simulink model "Analisis_dos_tanques"  (R2019a)
settings: Solver=VariableStepAuto  StartTime=0.0  StopTime=8000  RelTol=1e-3
values from neighbouring files (symbols this model uses):
  A1 = 95.5200    (= 95.52)    [Cluster_Discrimin.m]
  A2 = 64    [Cluster_Discrimin.m]
  k1 = 0.95800    (= 0.958)    [Cluster_Discrimin.m]
  k2 = 1.363500    (= 1.3635)    [Cluster_Discrimin.m]
undefined symbols (not defined in the file or in its folder): errortub, perturbacion, perturbacion2
settings Model: Creator=jalil  LastModifiedBy=david
settings DebuggingCC: ArithmeticOperatorsInVariantConditions=warning

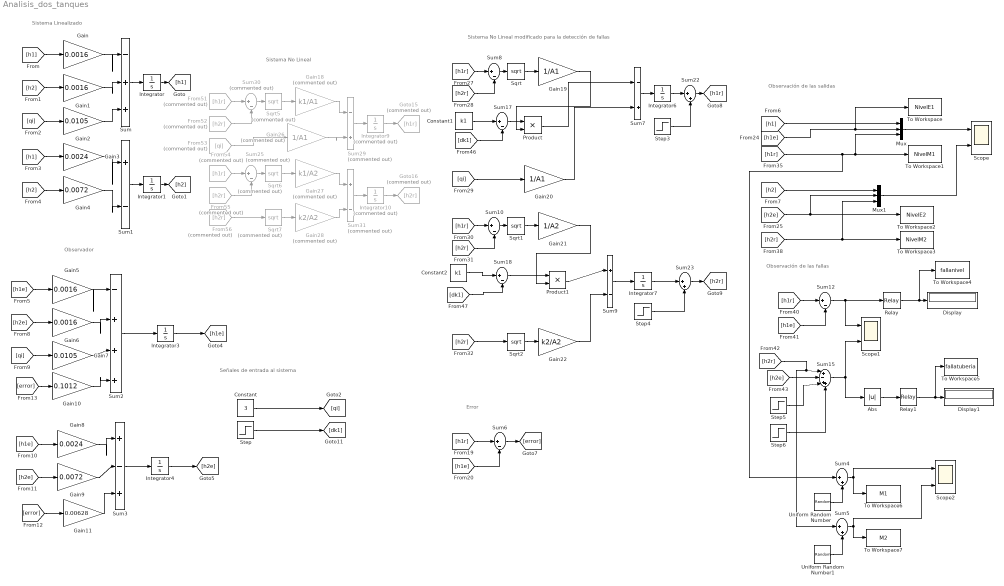
== system Analisis_dos_tanques ==
  note: Observador
  note: Sistema No Lineal modificado para la detección de fallas
  note: Sistema Linealizado
  note: Señales de entrada al sistema
  note: Observación de las salidas
  note: Error
  note: Sistema No Lineal
  note: Observación de las fallas
  Abs : Abs
  Constant : Constant  Value=3
  Constant1 : Constant  Value=k1
  Constant2 : Constant  Value=k1
  Display : Display
  Display1 : Display
  From51 : From  Commented=on  GotoTag=h1r
  From52 : From  Commented=on  GotoTag=h2r
  From53 : From  Commented=on  GotoTag=qi
  From54 : From  Commented=on  GotoTag=h1r
  From55 : From  Commented=on  GotoTag=h2r
  From56 : From  Commented=on  GotoTag=h2r
  Gain{,1,5..6} (4 alike) : Gain  Gain=0.0016
  Gain10 : Gain  Gain=0.1012
  Gain11 : Gain  Gain=0.00628
  Gain18 : Gain  Commented=on  Gain=k1/A1
  Gain19 : Gain  Gain=1/A1
  Gain2 : Gain  Gain=0.0105
  Gain20 : Gain  Gain=1/A1
  Gain21 : Gain  Gain=1/A2
  Gain22 : Gain  Gain=k2/A2
  Gain26 : Gain  Commented=on  Gain=1/A1
  Gain27 : Gain  Commented=on  Gain=k1/A2
  Gain28 : Gain  Commented=on  Gain=k2/A2
  Gain3 : Gain  Gain=0.0024
  Gain4 : Gain  Gain=0.0072
  Gain7 : Gain  Gain=0.0105
  Gain8 : Gain  Gain=0.0024
  Gain9 : Gain  Gain=0.0072
  Goto15 : Goto  Commented=on  GotoTag=h1r
  Goto16 : Goto  Commented=on  GotoTag=h2r
  Integrator{,1,6..7} (4 alike) : Integrator
  Integrator10 : Integrator  Commented=on
  Integrator3 : Integrator  InitialCondition=1
  Integrator4 : Integrator  InitialCondition=-1
  Integrator9 : Integrator  Commented=on
  Mux : Mux  Inputs=3
  Mux1 : Mux  Inputs=3
  Product : Product
  Product1 : Product
  Relay : Relay  OnSwitchValue=1.5  OffSwitchValue=-1000
  Relay1 : Relay  OnSwitchValue=1  OffSwitchValue=-1000
  Scope : Scope  NumInputPorts=2
  Scope1 : Scope  NumInputPorts=2
  Scope2 : Scope  NumInputPorts=2
  Sqrt : Sqrt  SaturateOnIntegerOverflow=on
  Sqrt1 : Sqrt  SaturateOnIntegerOverflow=on
  Sqrt2 : Sqrt  SaturateOnIntegerOverflow=on
  Sqrt5 : Sqrt  Commented=on  SaturateOnIntegerOverflow=on
  Sqrt6 : Sqrt  Commented=on  SaturateOnIntegerOverflow=on
  Sqrt7 : Sqrt  Commented=on  SaturateOnIntegerOverflow=on
  Step : Step  Time=3  After=errortub  SampleTime=0
  Step3 : Step  Time=5000  After=perturbacion  SampleTime=0
  Step4 : Step  Time=3000  After=perturbacion2  SampleTime=0
  Step5 : Step  Time=0  After=-0.6  SampleTime=0
  Step6 : Step  Time=300  After=0.6  SampleTime=0
  Sum : Sum  Inputs=|-++
  Sum{1,6,8..10,12,17..18} (8 alike) : Sum  Inputs=|+-
  Sum15 : Sum  Inputs=|+-++
  Sum2 : Sum  Inputs=|-+++
  Sum{4..5,22..23} (4 alike) : Sum  Inputs=|++
  Sum25 : Sum  Commented=on  Inputs=|+-
  Sum29 : Sum  Commented=on  Inputs=|-+
  Sum3 : Sum  Inputs=|+-+
  Sum30 : Sum  Commented=on  Inputs=|+-
  Sum31 : Sum  Commented=on  Inputs=|+-
  Sum7 : Sum  Inputs=|-+
  To Workspace : ToWorkspace  VariableName=NivelE1  SaveFormat=Timeseries  SampleTime=-1
      settings: Save2DSignal=2-D array (concatenate along first dimension)
  To Workspace1 : ToWorkspace  VariableName=NivelM1  SaveFormat=Timeseries  SampleTime=-1
      settings: Save2DSignal=2-D array (concatenate along first dimension)
  To Workspace2 : ToWorkspace  VariableName=NivelE2  SaveFormat=Timeseries  SampleTime=-1
      settings: Save2DSignal=2-D array (concatenate along first dimension)
  To Workspace3 : ToWorkspace  VariableName=NivelM2  SaveFormat=Timeseries  SampleTime=-1
      settings: Save2DSignal=2-D array (concatenate along first dimension)
  To Workspace4 : ToWorkspace  VariableName=fallanivel  SaveFormat=Timeseries  SampleTime=-1
      settings: Save2DSignal=2-D array (concatenate along first dimension)
  To Workspace5 : ToWorkspace  VariableName=fallatuberia  SaveFormat=Timeseries  SampleTime=-1
      settings: Save2DSignal=2-D array (concatenate along first dimension)
  To Workspace6 : ToWorkspace  VariableName=M1  SaveFormat=Timeseries  SampleTime=-1
      settings: Save2DSignal=2-D array (concatenate along first dimension)
  To Workspace7 : ToWorkspace  VariableName=M2  SaveFormat=Timeseries  SampleTime=-1
      settings: Save2DSignal=2-D array (concatenate along first dimension)
  Uniform Random Number : UniformRandomNumber  Minimum=-3  Maximum=3
  Uniform Random Number1 : UniformRandomNumber  Minimum=-3  Maximum=3
  wires:
  [h1] -> Gain/1
  Gain/1 -> Sum/1
  [h2] -> Gain1/1
  Gain1/1 -> Sum/2
  [qi] -> Gain2/1
  Gain2/1 -> Sum/3
  Sum/1 -> Integrator/1
  Integrator/1 -> [h1]
  Integrator1/1 -> [h2]
  Sum1/1 -> Integrator1/1
  Gain4/1 -> Sum1/2
  [h2] -> Gain4/1
  Gain3/1 -> Sum1/1
  [h1] -> Gain3/1
  Constant/1 -> [qi]
  Integrator4/1 -> [h2e]
  Integrator3/1 -> [h1e]
  [h1r] -> Sum6/1
  [h1e] -> Sum6/2
  Sum6/1 -> [error]
  Mux/1 -> Scope/1
  Mux1/1 -> Scope/2
  [h1] -> Mux/1
  [h2] -> Mux1/1
  [h1e] -> To Workspace/1, Mux/2
  [h2e] -> To Workspace2/1, Mux1/2
  Sum7/1 -> Integrator6/1
  [h2r] -> Sum8/2
  [h1r] -> Sum8/1
  Sum8/1 -> Sqrt/1
  Sqrt/1 -> Gain19/1
  [qi] -> Gain20/1
  Gain20/1 -> Sum7/2
  Sum9/1 -> Integrator7/1
  Sum10/1 -> Sqrt1/1
  [h2r] -> Sum10/2
  Sqrt1/1 -> Gain21/1
  [h1r] -> Sum10/1
  Sqrt2/1 -> Gain22/1
  [h2r] -> To Workspace3/1, Mux1/3
  [h1e] -> Sum12/2
  [h1r] -> Sum12/1
  [h2e] -> Sum15/2
  [h2r] -> Sum5/1, Sum15/1
  Sum12/1 -> Relay/1, Scope1/1
  Constant1/1 -> Sum17/1
  [dk1] -> Sum17/2
  Sum17/1 -> Product/1
  Gain19/1 -> Product/2
  Product/1 -> Sum7/1
  Gain21/1 -> Product1/2
  Product1/1 -> Sum9/1
  Sum18/1 -> Product1/1
  [dk1] -> Sum18/2
  Constant2/1 -> Sum18/1
  Step/1 -> [dk1]
  Integrator6/1 -> Sum22/1
  Step3/1 -> Sum22/2
  Sum22/1 -> [h1r]
  Integrator7/1 -> Sum23/1
  Step4/1 -> Sum23/2
  Sum23/1 -> [h2r]
  Gain28/1 -> Sum31/2
  Sum30/1 -> Sqrt5/1
  Sqrt7/1 -> Gain28/1
  Integrator10/1 -> Goto16/1
  From56/1 -> Sqrt7/1
  From54/1 -> Sum25/1
  Gain27/1 -> Sum31/1
  Sum31/1 -> Integrator10/1
  Gain18/1 -> Sum29/1
  Sqrt5/1 -> Gain18/1
  Sqrt6/1 -> Gain27/1
  Integrator9/1 -> Goto15/1
  From53/1 -> Gain26/1
  Sum29/1 -> Integrator9/1
  From51/1 -> Sum30/1
  Gain26/1 -> Sum29/2
  From55/1 -> Sum25/2
  From52/1 -> Sum30/2
  Sum25/1 -> Sqrt6/1
  [h1e] -> Gain8/1
  Gain6/1 -> Sum2/2
  [qi] -> Gain7/1
  Gain5/1 -> Sum2/1
  Gain8/1 -> Sum3/1
  [h2e] -> Gain6/1
  Gain7/1 -> Sum2/3
  [h2e] -> Gain9/1
  Sum2/1 -> Integrator3/1
  Sum3/1 -> Integrator4/1
  [h1e] -> Gain5/1
  Gain9/1 -> Sum3/2
  [error] -> Gain10/1
  Gain10/1 -> Sum2/4
  [error] -> Gain11/1
  Gain11/1 -> Sum3/3
  Gain22/1 -> Sum9/2
  [h2r] -> Sqrt2/1
  Relay/1 -> To Workspace4/1, Display/1
  Relay1/1 -> To Workspace5/1, Display1/1
  Sum15/1 -> Scope1/2, Abs/1
  Step5/1 -> Sum15/3
  Step6/1 -> Sum15/4
  Abs/1 -> Relay1/1
  [h1r] -> Sum4/1, To Workspace1/1, Mux/3
  Uniform Random Number/1 -> Sum4/2
  Sum4/1 -> To Workspace6/1, Scope2/1
  Uniform Random Number1/1 -> Sum5/2
  Sum5/1 -> Scope2/2, To Workspace7/1
